simulink model "robot"  (R2016b)
settings: Solver=ode3  StartTime=0.0  StopTime=inf  RelTol=1e-3  EnableMultiTasking=on
libraries: vexarmcortexlib x18
settings Model: ExtModeTrigDuration=25  Creator=Chase  LastModifiedBy=Chase
settings DataIOCC: LimitDataPoints=on  SignalLoggingSaveFormat=ModelDataLogs
settings OptimizationCC: ExpressionDepthLimit=2147483647  LifeSpan=Inf  MaxStackSize=64
settings DebuggingCC: UnderspecifiedInitializationDetection=Classic  MergeDetectMultiDrivingBlocksExec=none  InheritedTsInSrcMsg=none  FcnCallInpInsideContextMsg=warning  UnconnectedInputMsg=none  UnconnectedOutputMsg=none  StateNameClashWarn=warning  SFUnexpectedBacktrackingDiag=warning  SFNoUnconditionalDefaultTransitionDiag=warning  SFExecutionAtInitializationDiag=none
settings HardwareCC: ProdBitPerPointer=32  ProdBitPerSizeT=32  ProdBitPerPtrDiffT=32  ProdLargestAtomicInteger=Long  ProdLargestAtomicFloat=Double  ProdIntDivRoundTo=Undefined  ProdWordSize=32  ProdHWDeviceType=ARM Compatible->ARM Cortex
settings ModelReferenceCC: PropagateSignalLabelsOutOfModel=off
settings RTWCC: SystemTargetFile=ert.tlc  HardwareBoard=ARM Cortex-based VEX Microcontroller  TemplateMakefile=ert_default_tmf  Description=Embedded Coder  Toolchain=GNU Tools for VEX ARM Cortex
settings CodeAppCC: IgnoreCustomStorageClasses=off  CustomSymbolStrType=$N$R$M  InternalIdentifier=Classic
settings ERTTargetCC: CodeReplacementLibrary=GCC ARM Cortex-M3  ConvertIfToSwitch=off  SuppressUnreachableDefaultCases=off

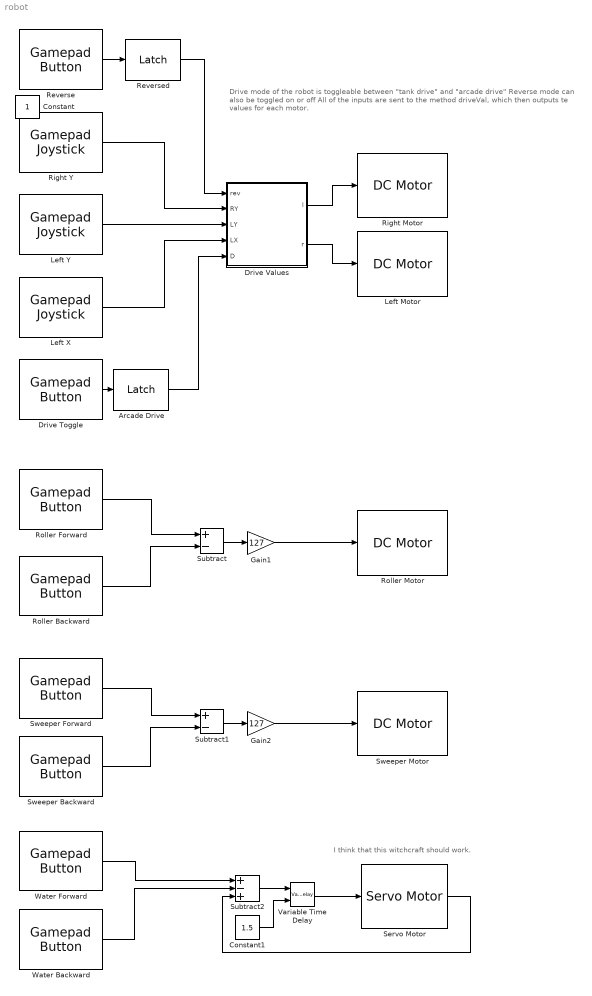
== system robot ==
  note: I think that this witchcraft should work.
  note: Drive mode of the robot is toggleable between "tank drive" and "arcade drive"
      |
      | Reverse mode can also be toggled on or off
      |
      | All of the inputs are sent to the method driveVal, which then outputs te values for each motor.
  Arcade Drive : vexarmcortexlib/Utilities/Latch  output0=off
  Constant1 : Constant  Value=1.5
  Drive Toggle : vexarmcortexlib/Gamepad Button  joystick=1  chan=6  button56=Up  button78=Right  SimulationIn=off  sample_time=0.2
  Drive Values : MATLAB Function  TreatAsAtomicUnit=on
      settings: CopyFcn=set_param(gcb, 'LinkStatus', 'none') ;
  Gain1 : Gain  Gain=127
  Gain2 : Gain  Gain=127
  Left Motor : vexarmcortexlib/DC Motor  motor=3  scaleFactor=1/13.5  SimulationOut=off
  Left X : vexarmcortexlib/Gamepad Joystick  joystick=1  chan=4  SimulationIn=off  sample_time=0.2
  Left Y : vexarmcortexlib/Gamepad Joystick  joystick=1  chan=3  SimulationIn=off  sample_time=0.2
  Reverse : vexarmcortexlib/Gamepad Button  joystick=1  chan=5  button56=Up  button78=Right  SimulationIn=off  sample_time=0.2
  Reversed : vexarmcortexlib/Utilities/Latch  output0=off
  Right Motor : vexarmcortexlib/DC Motor  motor=2  scaleFactor=1/13.5  SimulationOut=off
  Right Y : vexarmcortexlib/Gamepad Joystick  joystick=1  chan=2  SimulationIn=off  sample_time=0.2
  Roller Backward : vexarmcortexlib/Gamepad Button  joystick=1  chan=7  button56=Up  button78=Down  SimulationIn=off  sample_time=0.2
  Roller Forward : vexarmcortexlib/Gamepad Button  joystick=1  chan=7  button56=Up  button78=Up  SimulationIn=off  sample_time=0.2
  Roller Motor : vexarmcortexlib/DC Motor  motor=3  scaleFactor=1/13.5  SimulationOut=off
  Servo Motor : vexarmcortexlib/Servo Motor  motor=6  scaleFactor=60/127  SimulationOut=on
  Subtract : Sum  Inputs=+-
  Subtract1 : Sum  Inputs=+-
  Subtract2 : Sum  Inputs=+-+
  Sweeper Backward : vexarmcortexlib/Gamepad Button  joystick=1  chan=8  button56=Up  button78=Down  SimulationIn=off  sample_time=0.2
  Sweeper Forward : vexarmcortexlib/Gamepad Button  joystick=1  chan=8  button56=Up  button78=Up  SimulationIn=off  sample_time=0.2
  Sweeper Motor : vexarmcortexlib/DC Motor  motor=5  scaleFactor=1/13.5  SimulationOut=off
  Variable Time Delay : VariableTransportDelay  MaximumDelay=10
  Water Backward : vexarmcortexlib/Gamepad Button  joystick=1  chan=8  button56=Up  button78=Left  SimulationIn=off  sample_time=0.2
  Water Forward : vexarmcortexlib/Gamepad Button  joystick=1  chan=8  button56=Up  button78=Right  SimulationIn=off  sample_time=0.2
  Constant : Constant  IOType=siggen
  wires:
  Reverse/1 -> Reversed/1
  Drive Toggle/1 -> Arcade Drive/1
  Roller Forward/1 -> Subtract/1
  Roller Backward/1 -> Subtract/2
  Subtract/1 -> Gain1/1
  Gain1/1 -> Roller Motor/1
  Subtract1/1 -> Gain2/1
  Sweeper Forward/1 -> Subtract1/1
  Sweeper Backward/1 -> Subtract1/2
  Gain2/1 -> Sweeper Motor/1
  Left Y/1 -> Drive Values/3(LY)
  Left X/1 -> Drive Values/4(LX)
  Arcade Drive/1 -> Drive Values/5(D)
  Right Y/1 -> Drive Values/2(RY)
  Reversed/1 -> Drive Values/1(rev)
  Drive Values/2(r) -> Left Motor/1
  Drive Values/1(l) -> Right Motor/1
  Water Forward/1 -> Subtract2/1
  Water Backward/1 -> Subtract2/2
  Servo Motor/1 -> Subtract2/3
  Subtract2/1 -> Variable Time Delay/1
  Variable Time Delay/1 -> Servo Motor/1
  Constant1/1 -> Variable Time Delay/2

== matlab function robot/Drive Values ==
  data: rev input; l output; RY input; LY input; LX input; D input; r output
function [l, r] = driveVal(rev, RY, LY, LX, D)
    if rev == 0
        rev = -1;
    end
    
    if D == 1   %# Drive mode is Arcade
        l = (RY + LX) * rev;
        r = (RY - LX) * rev;
    else        %# Drive mode is Tank
        l = LY * rev;
        r = RY * rev;
    end
end
